simulink model "oldVers"  (R2022a)
settings: Solver=ode1  StartTime=0.0  StopTime=1  FixedStep=0.000001  RelTol=1e-3
values from neighbouring files (symbols this model uses):
  Cm = 0.05    [matlab2.mat]
  Jm = 1    [matlab2.mat]
  k_eq = 1    [matlab2.mat]
  k_pos = 1    [matlab2.mat]
  Ki_Curr = 1666    [matlab2.mat]
  Kinv = 18    [matlab2.mat]
  Kp_Curr = 0.0229017    [matlab2.mat]
  Re = 0.357267    [matlab2.mat]
  T_eq = 0.00052    [matlab2.mat]
  T_eq2 = 0.0018    [matlab2.mat]
  Te = 0.0006    [matlab2.mat]
  Tinv = 0.00026    [matlab2.mat]
libraries: simulink x2
settings Model: Creator=Ruslan  LastModifiedBy=Ruslan
settings SolverCC: AlgebraicLoopSolver=TrustRegion
settings DebuggingCC: SFMachineParentedDataDiag=warning
settings RTWCC: DLArmComputeVersion=19.05

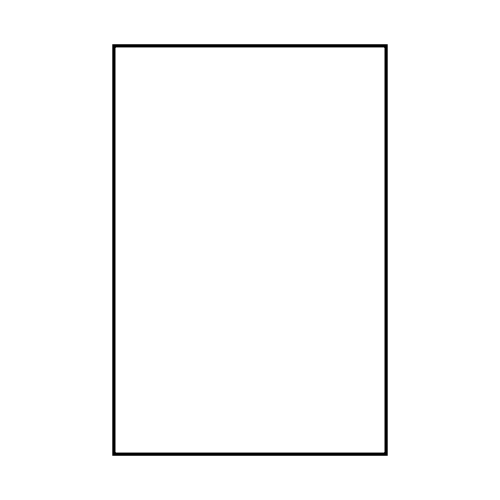
[thumbnail: Simulink's stored preview of the top-level diagram]
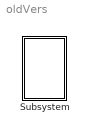
== system oldVers ==
  Subsystem : Subsystem

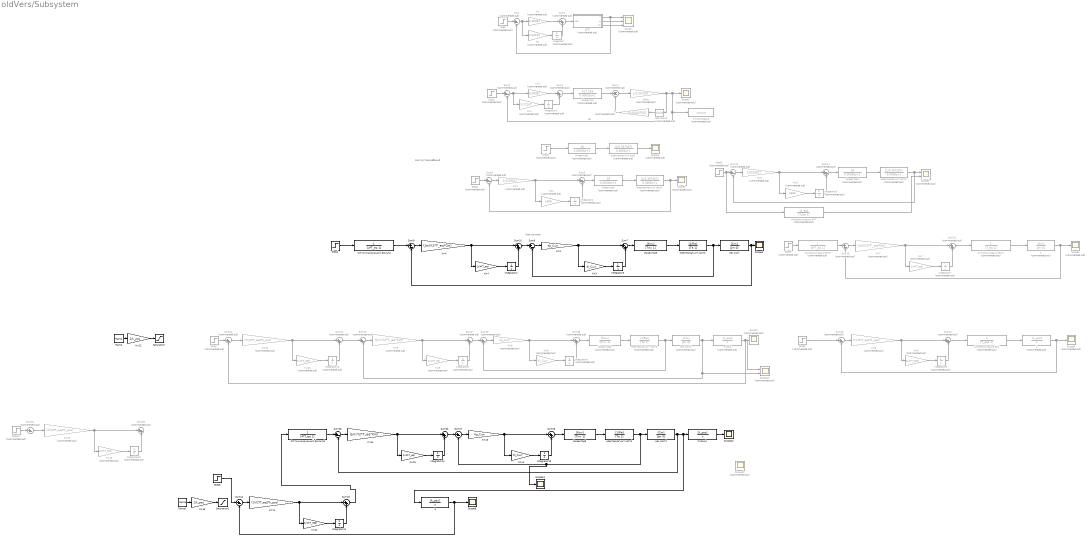
== system oldVers/Subsystem ==
  note: Контур тока
  note: Контур тока рабочий
  1 : TransferFcn  Commented=on  Numerator=[Cm]  Denominator=[Jm 0]
  1/Rяц : Gain  Commented=on  Gain=1/0.357267
  2 : TransferFcn  Commented=on  Numerator=[k_pos]  Denominator=[1 0]
  3 : TransferFcn  Numerator=[k_pos]  Denominator=[1 0]
  Derivative : Derivative  Commented=on
  Integrator{,1..2,5..10,12} (10 alike) : Integrator  Commented=on
  Integrator{3..4,11,13..14} (5 alike) : Integrator
  Kп : Gain  Commented=on  Gain=0.00067
  Kп1 : Gain  Commented=on  Gain=0.00067
  Kп10 : Gain  Commented=on  Gain=(1)/(2*T_eq2*k_pos)
  Kп11 : Gain  Gain=(1)/(2*T_eq2*k_pos)
  Kп12 : Gain  Commented=on  Gain=(1)/(2*T_eq2*k_pos)
  Kп13 : Gain  Gain=Kp_Curr
  Kп14 : Gain  Gain=(Jm)/(2*T_eq*Cm)
  Kп2 : Gain  Commented=on  Gain=0.0229017
  Kп3 : Gain  Gain=Kp_Curr
  Kп4 : Gain  Gain=(Jm)/(2*T_eq*Cm)
  Kп5 : Gain  Commented=on  Gain=0.0229017
  Kп6 : Gain  Commented=on  Gain=(1)/(2*T_eq2*k_pos)
  Kп7 : Gain  Commented=on  Gain=(Jm)/(2*T_eq*Cm)
  Kп8 : Gain  Commented=on  Gain=Kp_Curr
  Kп9 : Gain  Commented=on  Gain=(Jm)/(2*T_eq*Cm)
  L : Gain  Commented=on  Gain=0.001457602
  Ramp : simulink/Sources/Ramp  slope=50  start=0  InitialOutput=0
  Ramp1 : simulink/Sources/Ramp  slope=120  start=0  InitialOutput=0
  Saturation : Saturate  UpperLimit=96  LowerLimit=-40
  Saturation1 : Saturate  UpperLimit=96  LowerLimit=-40
  Scope : Scope  Commented=on  NumInputPorts=3
  Scope{1..3,6..7,9} (6 alike) : Scope  Commented=on
  Scope10 : Scope  Commented=on  NumInputPorts=2
  Scope11 : Scope  Commented=on  NumInputPorts=2
  Scope{4,8,12..13} (4 alike) : Scope
  Scope5 : Scope  Commented=on  NumInputPorts=2
  Step : Step  Commented=on  Time=0  After=-12  SampleTime=0
  Step{1..3,5..7,9..10} (8 alike) : Step  Commented=on  Time=0  SampleTime=0
  Step4 : Step  Time=0  SampleTime=0
  Step8 : Step  Time=0  SampleTime=0
  Sum{,2,6,12,15..16,19..20,22,30} (10 alike) : Sum  Commented=on  Inputs=|+-
  Sum{1,3,5,11,13..14,17..18,21,29} (10 alike) : Sum  Commented=on  Inputs=|++
  Sum{7,10,23,25..26} (5 alike) : Sum  Inputs=|++
  Sum{8..9,24,27..28} (5 alike) : Sum  Inputs=|+-
  Sum4 : Sum  Commented=on  Inputs=-+-
  To Workspace : ToWorkspace  Commented=on  VariableName=simout  SaveFormat=Timeseries  SampleTime=-1
  Аппроксимация ЗКС : TransferFcn  Commented=on  Denominator=[T_eq2 1]
  Аппроксимация ЗКТ : TransferFcn  Commented=on  Numerator=[k_eq]  Denominator=[T_eq 1]
  Аппроксимация ЗКТ1 : TransferFcn  Commented=on  Denominator=[T_eq 1]
  Аппроксимация ЗКТ3 : TransferFcn  Commented=on  Denominator=[4*T_eq 1]
  ДПТ : Subsystem  Commented=on
  Инвентор : TransferFcn  Commented=on  Numerator=[617.143]  Denominator=[0.00026 1]
  Инвентор1 : TransferFcn  Commented=on  Numerator=[18]  Denominator=[0.00026 1]
  Инвентор2 : TransferFcn  Commented=on  Numerator=[18]  Denominator=[0.00026 1]
  Инвентор3 : TransferFcn  Numerator=[Kinv]  Denominator=[Tinv 1]
  Инвентор4 : TransferFcn  Commented=on  Numerator=[18]  Denominator=[0.00026 1]
  Инвентор5 : TransferFcn  Numerator=[Kinv]  Denominator=[Tinv 1]
  Инвентор6 : TransferFcn  Commented=on  Numerator=[Kinv]  Denominator=[Tinv 1]
  Ки : Gain  Commented=on  Gain=0.22167
  Ки1 : Gain  Commented=on  Gain=0.22167
  Ки10 : Gain  Commented=on  Gain=1/(4*T_eq2)
  Ки11 : Gain  Gain=1/(4*T_eq2)
  Ки12 : Gain  Gain=1/k_pos
  Ки13 : Gain  Commented=on  Gain=1/(4*T_eq2)
  Ки14 : Gain  Gain=Ki_Curr
  Ки15 : Gain  Gain=1/(4*T_eq)
  Ки16 : Gain  Gain=1/k_pos
  Ки2 : Gain  Commented=on  Gain=1666
  Ки3 : Gain  Gain=Ki_Curr
  Ки4 : Gain  Gain=1/(4*T_eq)
  Ки5 : Gain  Commented=on  Gain=1666
  Ки6 : Gain  Commented=on  Gain=1/(4*T_eq2)
  Ки7 : Gain  Commented=on  Gain=1/(4*T_eq)
  Ки8 : Gain  Commented=on  Gain=Ki_Curr
  Ки9 : Gain  Commented=on  Gain=1/(4*T_eq)
  Оптимизирующий фильтр : TransferFcn  Denominator=[4*T_eq 1]
  Оптимизирующий фильтр1 : TransferFcn  Denominator=[4*T_eq 1]
  мех сост : TransferFcn  Numerator=[Cm]  Denominator=[Jm 0]
  мех сост1 : TransferFcn  Numerator=[Cm]  Denominator=[Jm 0]
  мех сост2 : TransferFcn  Commented=on  Numerator=[Cm]  Denominator=[Jm 0]
  полож : TransferFcn  Commented=on  Numerator=[k_pos]  Denominator=[1 0]
  полож1 : TransferFcn  Numerator=[k_pos]  Denominator=[1 0]
  электромагнит сост : TransferFcn  Commented=on  Numerator=[1/0.357267]  Denominator=[0.0006 1]
  электромагнит сост1 : TransferFcn  Commented=on  Numerator=[1/0.357267]  Denominator=[0.0006 1]
  электромагнит сост2 : TransferFcn  Numerator=[1/Re]  Denominator=[Te 1]
  электромагнит сост3 : TransferFcn  Commented=on  Numerator=[1/0.357267]  Denominator=[0.0006 1]
  электромагнит сост4 : TransferFcn  Numerator=[1/Re]  Denominator=[Te 1]
  электромагнит сост5 : TransferFcn  Commented=on  Numerator=[1/Re]  Denominator=[Te 1]
  wires:
  Sum/1 -> Kп/1, Ки/1
  Sum1/1 -> ДПТ/1(Uвх)
  Ки/1 -> Integrator/1
  Step/1 -> Sum/1
  Kп/1 -> Sum1/1
  ДПТ/1(I) -> Sum/2, Scope/1
  ДПТ/3(M) -> Scope/3
  Integrator/1 -> Sum1/2
  ДПТ/2(ω) -> Scope/2
  Integrator1/1 -> Sum3/2
  Sum2/1 -> Kп1/1, Ки1/1
  Kп1/1 -> Sum3/1
  Ки1/1 -> Integrator1/1
  Step1/1 -> Sum2/1
  Sum4/1 -> 1/Rяц/1
  L/1 -> Sum4/3
  Derivative/1 -> L/1
  1/Rяц/1 -> Derivative/1, To Workspace/1, Sum2/2, Scope2/1  "Iя"
  Sum3/1 -> Инвентор/1
  Инвентор/1 -> Sum4/2
  Step2/1 -> Инвентор1/1
  Инвентор1/1 -> электромагнит сост/1
  электромагнит сост/1 -> Scope1/1
  Инвентор2/1 -> электромагнит сост1/1
  электромагнит сост1/1 -> Scope3/1, Sum6/2
  Ки2/1 -> Integrator2/1
  Integrator2/1 -> Sum5/2
  Kп2/1 -> Sum5/1, Ки2/1
  Sum5/1 -> Инвентор2/1
  Step3/1 -> Sum6/1
  Sum6/1 -> Kп2/1
  Kп3/1 -> Sum7/1, Ки3/1
  Integrator3/1 -> Sum7/2
  Sum8/1 -> Kп3/1
  электромагнит сост2/1 -> мех сост/1, Sum8/2
  Инвентор3/1 -> электромагнит сост2/1
  Sum7/1 -> Инвентор3/1
  Ки3/1 -> Integrator3/1
  Kп4/1 -> Ки4/1, Sum10/1
  Integrator4/1 -> Sum10/2
  Ки4/1 -> Integrator4/1
  Sum9/1 -> Kп4/1
  Sum10/1 -> Sum8/1
  мех сост/1 -> Sum9/2, Scope4/1
  Kп5/1 -> Sum11/1, Ки5/1
  Integrator5/1 -> Sum11/2
  Sum12/1 -> Kп5/1
  Step5/1 -> Аппроксимация ЗКТ/1, Sum12/1
  электромагнит сост3/1 -> Scope5/1, Sum12/2
  Инвентор4/1 -> электромагнит сост3/1
  Sum11/1 -> Инвентор4/1
  Ки5/1 -> Integrator5/1
  Аппроксимация ЗКТ/1 -> Scope5/2
  Ки9/1 -> Integrator9/1
  Integrator9/1 -> Sum17/2
  Kп9/1 -> Ки9/1, Sum17/1
  Sum20/1 -> Kп9/1
  мех сост2/1 -> Scope10/2, Sum20/2, полож/1
  Integrator8/1 -> Sum18/2
  Sum19/1 -> Kп8/1
  Sum17/1 -> Sum19/1
  Kп8/1 -> Sum18/1, Ки8/1
  Инвентор6/1 -> электромагнит сост5/1
  Sum18/1 -> Инвентор6/1
  электромагнит сост5/1 -> мех сост2/1, Sum19/2
  Ки8/1 -> Integrator8/1
  Integrator10/1 -> Sum21/2
  Kп10/1 -> Ки10/1, Sum21/1
  Ки10/1 -> Integrator10/1
  полож/1 -> Sum22/2, Scope10/1, Scope7/1
  Sum22/1 -> Kп10/1
  Ки7/1 -> Integrator7/1
  Sum13/1 -> Аппроксимация ЗКТ1/1
  Kп7/1 -> Ки7/1, Sum13/1
  Sum16/1 -> Kп7/1
  Аппроксимация ЗКТ1/1 -> 1/1
  Integrator7/1 -> Sum13/2
  1/1 -> Scope6/1, Sum16/2
  Step6/1 -> Аппроксимация ЗКТ3/1
  Аппроксимация ЗКТ3/1 -> Sum16/1
  Step4/1 -> Оптимизирующий фильтр/1
  Оптимизирующий фильтр/1 -> Sum9/1
  2/1 -> Scope9/1, Sum15/2
  Sum14/1 -> Аппроксимация ЗКС/1
  Ки6/1 -> Integrator6/1
  Kп6/1 -> Ки6/1, Sum14/1
  Sum15/1 -> Kп6/1
  Integrator6/1 -> Sum14/2
  Step9/1 -> Sum15/1
  Аппроксимация ЗКС/1 -> 2/1
  Ramp/1 -> Ки12/1
  Ки12/1 -> Saturation/1
  Sum21/1 -> Sum20/1
  Step7/1 -> Sum22/1
  Kп11/1 -> Ки11/1, Sum23/1
  Sum24/1 -> Kп11/1
  Sum23/1 -> Оптимизирующий фильтр1/1
  3/1 -> Scope8/1, Sum24/2
  Integrator11/1 -> Sum23/2
  Ки11/1 -> Integrator11/1
  мех сост1/1 -> Sum28/2, 3/1, полож1/1
  Sum28/1 -> Kп14/1
  Step10/1 -> Sum30/1
  Инвентор5/1 -> электромагнит сост4/1
  электромагнит сост4/1 -> мех сост1/1, Scope13/1, Sum27/2
  Kп14/1 -> Ки15/1, Sum25/1
  Ки13/1 -> Integrator12/1
  Ки14/1 -> Integrator13/1
  Integrator13/1 -> Sum26/2
  Integrator12/1 -> Sum29/2
  Sum26/1 -> Инвентор5/1
  Sum27/1 -> Kп13/1
  Kп13/1 -> Sum26/1, Ки14/1
  Integrator14/1 -> Sum25/2
  Sum25/1 -> Sum27/1
  Sum30/1 -> Kп12/1
  полож1/1 -> Scope12/1
  Ки15/1 -> Integrator14/1
  Kп12/1 -> Ки13/1, Sum29/1
  Ки16/1 -> Saturation1/1
  Ramp1/1 -> Ки16/1
  Оптимизирующий фильтр1/1 -> Sum28/1
  Step8/1 -> Sum24/1

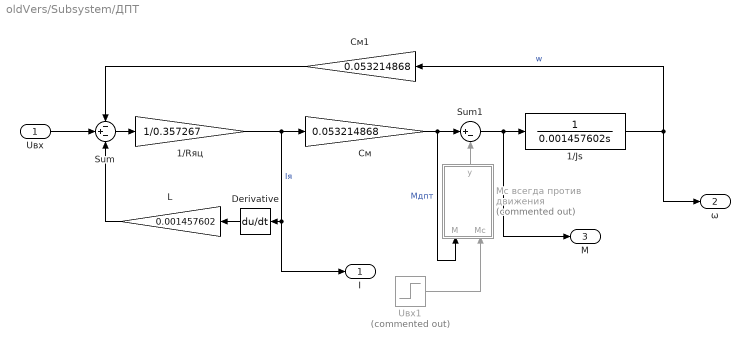
== system oldVers/Subsystem/ДПТ ==
  Uвх : Inport
  1/Js : TransferFcn  Denominator=[0.001457602 0]
  1/Rяц : Gain  Gain=1/0.357267
  Cм : Gain  Gain=0.053214868
  Cм1 : Gain  Gain=0.053214868
  Derivative : Derivative
  L : Gain  Gain=0.001457602
  Sum : Sum  Inputs=-+-
  Sum1 : Sum  Inputs=|+-
  Uвх1 : Step  Commented=on  After=0.06  SampleTime=0
  Мс всегда против движения : MATLAB Function  Commented=on  TreatAsAtomicUnit=on
  I : Outport
  ω : Outport  Port=2
  M : Outport  Port=3
  wires:
  1/Rяц/1 -> I/1, Derivative/1, Cм/1  "Iя"
  Uвх/1 -> Sum/2
  L/1 -> Sum/3
  1/Js/1 -> Cм1/1, ω/1  "w"
  Cм1/1 -> Sum/1
  Derivative/1 -> L/1
  Sum1/1 -> M/1, 1/Js/1
  Uвх1/1 -> Мс всегда против движения/2(Mc)
  Sum/1 -> 1/Rяц/1
  Cм/1 -> Мс всегда против движения/1(M), Sum1/1  "Мдпт"
  Мс всегда против движения/1(y) -> Sum1/2

== matlab function oldVers/Subsystem/ДПТ/Мс всегда против движения ==
  data: M input; Mc input; y output
function y = fcn(M, Mc)
if (M>0)
    y = Mc;
else
    y = -Mc;
end
